simulink model "simulink_tri_motor_drone"  (R2020a)
settings: Solver=VariableStepAuto  StartTime=0.0  StopTime=50  RelTol=1e-3
values from neighbouring files (symbols this model uses):
  airDensity = 1.225    [tri_drone.m]
  areaWheelFront = wheelHeight*wheelWidth    (= 0.004)    [tri_drone.m]
  areaWing = 0.121    [tri_drone.m]
  cDFront = 0.9    [tri_drone.m]
  cDtable = [0.174 0.157 0.141 0.127 0.113 0.100 0.088 0.077 0.067 0.058 0.051 0.044 0.038 0.033 0.028 0.025 0.023 0.021 0.020 0.020 0.021 0.023 0.026 0.029 0.033 0.038 0.043 0.050 0.056 0.064 0.072 0.081 0.091 0.101 0.112 0.124 0.137 0.150 0.165 0.180 0.196 0.212 0.229 0.245 0.261 0.277 0.292 0.306 0.319 0.331 0.341]    [tri_drone.m]
  cLtable = [-1.07 -1.02 -0.97 -0.92 -0.87 -0.81 -0.76 -0.70 -0.65 -0.59 -0.54 -0.48 -0.43 -0.37 -0.31 -0.25 -0.19 -0.13 -0.07 -0.01 0.05 0.11 0.17 0.23 0.29 0.35 0.40 0.46 0.52 0.57 0.63 0.68 0.74 0.79 0.85 0.90 0.95 1.00 1.05 1.10 1.15 1.20 1.25 1.29 1.32 1.36 1.38 1.41 1.43 1.44 1.45]    [tri_drone.m]
  heightRef = 1.0    (= 1)    [tri_drone.m]
  hoverRot = w(11)    [tri_drone.m]
  hoverVel = trustPerPropeller / Ktrust /pi * 180.0    [tri_drone.m]
  hoverVoltagefine = 0.35*11.9    (= 4.165)    [tri_drone.m]
  KDheightcoarse = 15.0    (= 15)    [tri_drone.m]
  KDheightfine = 0    [tri_drone.m]
  KDrag = 8 * (ampMax * Km / (rpmMax / 60 * 2 * pi))    (= 0.000150440801971)    [tri_drone.m]
  KIheightcoarse = 5.0    (= 5)    [tri_drone.m]
  KIheightfine = 0    [tri_drone.m]
  Km = 60/(Kv * 2 * pi)    (= 0.00415186808066)    [tri_drone.m]
  KPheightcoarse = 0.1    [tri_drone.m]
  KPheightfine = 0    [tri_drone.m]
  Ktrust = (trustMax * g)/(rpmMax / 60 * 2 * pi)    (= 0.00223215912077)    [tri_drone.m]
  mBodyTotal = 0.422 + mBattery    (= 0.797)    [tri_drone.m]
  motorMass = 0.022    [tri_drone.m]
  N = 1000000    [tri_drone.m]
  pitch_lower_limit = theta(1)    [tri_drone.m]
  pitch_upper_limit = theta(end)    [tri_drone.m]
  propellerMass = 0.012    [tri_drone.m]
  Ra = RaVolt/ampMax    (= 0.133333333333)    [tri_drone.m]
  rInner = armRadius    (= 0.27)    [tri_drone.m]
  rOuter = armRadius + wLength    (= 0.91)    [tri_drone.m]
  theta = [-10 -9.5 -9.0 -8.5 -8.0 -7.5 -7.0 -6.5 -6.0 -5.5 -5.0 -4.5 -4.0 -3.5 -3.0 -2.5 -2.0 -1.5 -1.0 -0.5 0 0.5 1.0 1.5 2.0 2.5 3.0 3.5 4.0 4.5 5.0 5.5 6.0 6.5 7.0 7.5 8.0 8.5 9.0 9.5 10.0 10.5 11.0 11.5 12.0 12.5 13.0 13.5 14.0 14.5 15.0]    [tri_drone.m]
  Ts = 0.002    [tri_drone.m]
  Ts2 = 0.03    [tri_drone.m]
  wHeight = 0.025    [tri_drone.m]
  wingDensity = 50    [tri_drone.m]
  wLength = 0.64    [tri_drone.m]
  wWidth = 0.20    (= 0.2)    [tri_drone.m]
undefined symbols (not defined in the file or in its folder): X, Y, Z
libraries: sm_lib x53, nesl_utility x45
(part 1 of 3)
settings Model: Creator=Jonas  LastModifiedBy=Jonas

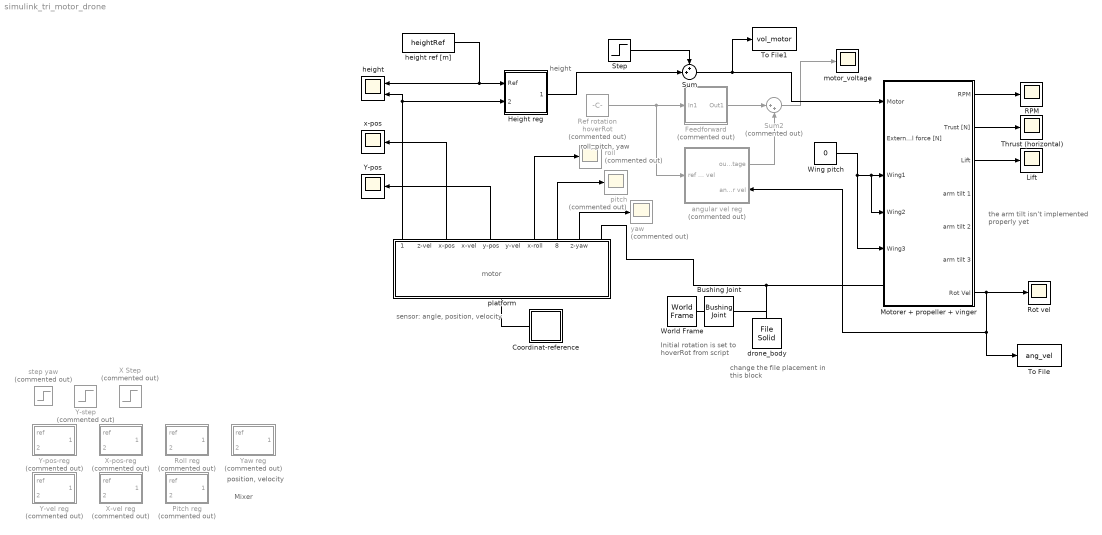
== system simulink_tri_motor_drone ==
  note: the arm tilt isn't implemented properly yet
  note: change the file placement in this block
  note: Initial rotation is set to
      | hoverRot from script
  note: roll, pitch, yaw
  note: position, velocity
  note: height
  note: motor
  note: Mixer
  note: sensor: angle, position, velocity
  Bushing Joint : sm_lib/Joints/Bushing Joint  JointMode=Normal  SenseConstraintForce=off  SenseConstraintForceX=off  SenseConstraintForceY=off  SenseConstraintForceZ=off  SenseConstraintTorque=off  SenseConstraintTorqueX=off  SenseConstraintTorqueY=off  SenseConstraintTorqueZ=off  SenseTotalForce=off  SenseTotalForceX=off  SenseTotalForceY=off  SenseTotalForceZ=off  SenseTotalTorque=off  SenseTotalTorqueX=off  SenseTotalTorqueY=off  SenseTotalTorqueZ=off  CompositeWrenchDir=FollowerOnBase  CompositeWrenchFrame=BaseFrame  PxEquilibriumPosition=0  PxEquilibriumPositionUnits=m  PxSpringStiffness=0  PxSpringStiffnessUnits=N/m  PxDampingCoefficient=0  PxDampingCoefficientUnits=N/(m/s)  PxTorqueActuationMode=NoTorque  PxMotionActuationMode=ComputedMotion  PxSensePosition=off  PxSenseVelocity=off  PxSenseAcceleration=off  PxSenseTorqueForce=off  PxSenseLowerLimitTorqueForce=off  PxSenseUpperLimitTorqueForce=off  PxLowerLimitSpecify=off  PxLowerLimitBound=-1  PxLowerLimitBoundUnits=m  PxLowerLimitStiffness=1e6  PxLowerLimitStiffnessUnits=N/m  PxLowerLimitDamping=1e3  PxLowerLimitDampingUnits=N/(m/s)  PxLowerLimitTransitionRegionWidth=1e-4  PxLowerLimitTransitionRegionWidthUnits=m  PxUpperLimitSpecify=off  PxUpperLimitBound=1  PxUpperLimitBoundUnits=m  PxUpperLimitStiffness=1e6  PxUpperLimitStiffnessUnits=N/m  PxUpperLimitDamping=1e3  PxUpperLimitDampingUnits=N/(m/s)  PxUpperLimitTransitionRegionWidth=1e-4  PxUpperLimitTransitionRegionWidthUnits=m  PxPositionTargetSpecify=off  PxPositionTargetPriority=High  PxPositionTargetValue=0  PxPositionTargetValueUnits=m  PxVelocityTargetSpecify=off  PxVelocityTargetPriority=High  PxVelocityTargetValue=0  PxVelocityTargetValueUnits=m/s  PyEquilibriumPosition=0  PyEquilibriumPositionUnits=m  PySpringStiffness=0  PySpringStiffnessUnits=N/m  PyDampingCoefficient=0  PyDampingCoefficientUnits=N/(m/s)  PyTorqueActuationMode=NoTorque  PyMotionActuationMode=ComputedMotion  PySensePosition=off  PySenseVelocity=off  PySenseAcceleration=off  PySenseTorqueForce=off  PySenseLowerLimitTorqueForce=off  PySenseUpperLimitTorqueForce=off  PyLowerLimitSpecify=off  PyLowerLimitBound=-1  PyLowerLimitBoundUnits=m  PyLowerLimitStiffness=1e6  PyLowerLimitStiffnessUnits=N/m  PyLowerLimitDamping=1e3  PyLowerLimitDampingUnits=N/(m/s)  PyLowerLimitTransitionRegionWidth=1e-4  PyLowerLimitTransitionRegionWidthUnits=m  PyUpperLimitSpecify=off  PyUpperLimitBound=1  PyUpperLimitBoundUnits=m  PyUpperLimitStiffness=1e6  PyUpperLimitStiffnessUnits=N/m  PyUpperLimitDamping=1e3  PyUpperLimitDampingUnits=N/(m/s)  PyUpperLimitTransitionRegionWidth=1e-4  PyUpperLimitTransitionRegionWidthUnits=m  PyPositionTargetSpecify=off  PyPositionTargetPriority=High  PyPositionTargetValue=0  PyPositionTargetValueUnits=m  PyVelocityTargetSpecify=off  PyVelocityTargetPriority=High  PyVelocityTargetValue=0  PyVelocityTargetValueUnits=m/s  PzEquilibriumPosition=0  PzEquilibriumPositionUnits=m  PzSpringStiffness=0  PzSpringStiffnessUnits=N/m  PzDampingCoefficient=0  PzDampingCoefficientUnits=N/(m/s)  PzTorqueActuationMode=NoTorque  PzMotionActuationMode=ComputedMotion  PzSensePosition=off  PzSenseVelocity=off  PzSenseAcceleration=off  PzSenseTorqueForce=off  PzSenseLowerLimitTorqueForce=off  PzSenseUpperLimitTorqueForce=off  PzLowerLimitSpecify=off  PzLowerLimitBound=-1  PzLowerLimitBoundUnits=m  PzLowerLimitStiffness=1e6  PzLowerLimitStiffnessUnits=N/m  PzLowerLimitDamping=1e3  PzLowerLimitDampingUnits=N/(m/s)  PzLowerLimitTransitionRegionWidth=1e-4  PzLowerLimitTransitionRegionWidthUnits=m  PzUpperLimitSpecify=off  PzUpperLimitBound=1  PzUpperLimitBoundUnits=m  PzUpperLimitStiffness=1e6  PzUpperLimitStiffnessUnits=N/m  PzUpperLimitDamping=1e3  PzUpperLimitDampingUnits=N/(m/s)  PzUpperLimitTransitionRegionWidth=1e-4  PzUpperLimitTransitionRegionWidthUnits=m  PzPositionTargetSpecify=off  PzPositionTargetPriority=High  PzPositionTargetValue=0  PzPositionTargetValueUnits=m  PzVelocityTargetSpecify=off  PzVelocityTargetPriority=High  PzVelocityTargetValue=0  PzVelocityTargetValueUnits=m/s  RxEquilibriumPosition=0  RxEquilibriumPositionUnits=deg  RxSpringStiffness=0  RxSpringStiffnessUnits=N*m/deg  RxDampingCoefficient=0  RxDampingCoefficientUnits=N*m/(deg/s)  RxTorqueActuationMode=NoTorque  RxMotionActuationMode=ComputedMotion  RxSensePosition=off  RxSenseVelocity=off  RxSenseAcceleration=off  RxSenseTorqueForce=off  RxSenseLowerLimitTorqueForce=off  RxSenseUpperLimitTorqueForce=off  RxLowerLimitSpecify=off  RxLowerLimitBound=-90  RxLowerLimitBoundUnits=deg  RxLowerLimitStiffness=1e4  RxLowerLimitStiffnessUnits=N*m/deg  RxLowerLimitDamping=10  RxLowerLimitDampingUnits=N*m/(deg/s)  RxLowerLimitTransitionRegionWidth=0.1  RxLowerLimitTransitionRegionWidthUnits=deg  RxUpperLimitSpecify=off  RxUpperLimitBound=90  RxUpperLimitBoundUnits=deg  RxUpperLimitStiffness=1e4  RxUpperLimitStiffnessUnits=N*m/deg  RxUpperLimitDamping=10  RxUpperLimitDampingUnits=N*m/(deg/s)  RxUpperLimitTransitionRegionWidth=0.1  RxUpperLimitTransitionRegionWidthUnits=deg  RxPositionTargetSpecify=off  RxPositionTargetPriority=High  RxPositionTargetValue=0  RxPositionTargetValueUnits=deg  RxVelocityTargetSpecify=off  RxVelocityTargetPriority=High  RxVelocityTargetValue=0  RxVelocityTargetValueUnits=deg/s  RyEquilibriumPosition=0  RyEquilibriumPositionUnits=deg  RySpringStiffness=0  RySpringStiffnessUnits=N*m/deg  RyDampingCoefficient=0  RyDampingCoefficientUnits=N*m/(deg/s)  RyTorqueActuationMode=NoTorque  RyMotionActuationMode=ComputedMotion  RySensePosition=off  RySenseVelocity=off  RySenseAcceleration=off  RySenseTorqueForce=off  RySenseLowerLimitTorqueForce=off  RySenseUpperLimitTorqueForce=off  RyLowerLimitSpecify=off  RyLowerLimitBound=-90  RyLowerLimitBoundUnits=deg  RyLowerLimitStiffness=1e4  RyLowerLimitStiffnessUnits=N*m/deg  RyLowerLimitDamping=10  RyLowerLimitDampingUnits=N*m/(deg/s)  RyLowerLimitTransitionRegionWidth=0.1  RyLowerLimitTransitionRegionWidthUnits=deg  RyUpperLimitSpecify=off  RyUpperLimitBound=90  RyUpperLimitBoundUnits=deg  RyUpperLimitStiffness=1e4  RyUpperLimitStiffnessUnits=N*m/deg  RyUpperLimitDamping=10  RyUpperLimitDampingUnits=N*m/(deg/s)  RyUpperLimitTransitionRegionWidth=0.1  RyUpperLimitTransitionRegionWidthUnits=deg  RyPositionTargetSpecify=off  RyPositionTargetPriority=High  RyPositionTargetValue=0  RyPositionTargetValueUnits=deg  RyVelocityTargetSpecify=off  RyVelocityTargetPriority=High  RyVelocityTargetValue=0  RyVelocityTargetValueUnits=deg/s  RzEquilibriumPosition=0  RzEquilibriumPositionUnits=deg  RzSpringStiffness=0  RzSpringStiffnessUnits=N*m/deg  RzDampingCoefficient=0  RzDampingCoefficientUnits=N*m/(deg/s)  RzTorqueActuationMode=NoTorque  RzMotionActuationMode=ComputedMotion  RzSensePosition=off  RzSenseVelocity=off  RzSenseAcceleration=off  RzSenseTorqueForce=off  RzSenseLowerLimitTorqueForce=off  RzSenseUpperLimitTorqueForce=off  RzLowerLimitSpecify=off  RzLowerLimitBound=-90  RzLowerLimitBoundUnits=deg  RzLowerLimitStiffness=1e4  RzLowerLimitStiffnessUnits=N*m/deg  RzLowerLimitDamping=10  RzLowerLimitDampingUnits=N*m/(deg/s)  RzLowerLimitTransitionRegionWidth=0.1  RzLowerLimitTransitionRegionWidthUnits=deg  RzUpperLimitSpecify=off  RzUpperLimitBound=90  RzUpperLimitBoundUnits=deg  RzUpperLimitStiffness=1e4  RzUpperLimitStiffnessUnits=N*m/deg  RzUpperLimitDamping=10  RzUpperLimitDampingUnits=N*m/(deg/s)  RzUpperLimitTransitionRegionWidth=0.1  RzUpperLimitTransitionRegionWidthUnits=deg  RzPositionTargetSpecify=off  RzPositionTargetPriority=High  RzPositionTargetValue=0  RzPositionTargetValueUnits=deg  RzVelocityTargetSpecify=on  RzVelocityTargetPriority=High  RzVelocityTargetValue=initRot  RzVelocityTargetValueUnits=rad/s
  Coordinat-reference : Subsystem
  Feedforward : Subsystem  Commented=on
  Height reg : Subsystem
  Lift : Scope
  Motorer + propeller + vinger : Subsystem
  Pitch reg : Subsystem  Commented=on
  RPM : Scope
  Ref rotation : Constant  Commented=on  Value=hoverRot
  Roll reg : Subsystem  Commented=on
  Rot vel : Scope
  Step : Step  Time=25  After=0.39*11.9  SampleTime=0
  Sum : Sum  Inputs=++|
  Sum2 : Sum  Commented=on  Inputs=|++
  Thrust (horizontal) : Scope
  To File : ToFile  Filename=ang_vel
  To File1 : ToFile  Filename=vol_motor
  Wing pitch : Constant  Value=0
  World Frame : sm_lib/Frames and Transforms/World Frame
  X Step : Step  Commented=on  Time=1.5  After=0  SampleTime=0
  X-pos-reg : Subsystem  Commented=on
  X-vel reg : Subsystem  Commented=on
  Y-pos : Scope
  Y-pos-reg : Subsystem  Commented=on
  Y-step : Step  Commented=on  After=0  SampleTime=0
  Y-vel reg : Subsystem  Commented=on
  "Yaw reg " : Subsystem  Commented=on
  angular vel reg : Subsystem  Commented=on
      settings: PortSchema="{\"entries\":[{\"content\":{\"sides\":[{\"content\":{\"connectorIds\":[\"In1\"]},\"type\":\"ConnectorPlacement.EquallySpacedRectSide\",\"uuid\":\"77c843f2-849e-4254-8ab0-e659ee2bffc0\"},{\"content\":{\"connectorIds\":[\"Out1\",\"In2\"],\"side\":\"RIGHT\"},\"type\":\"ConnectorPlacement.EquallySpacedRectSide\",\"uuid\":\"827c0fe3-5880-493e-8320-005b0a787497\"},{\"content\":{\"connectorIds\":[],\"side\":\"TOP\"},\"type\":\"ConnectorPlacement.EquallySpacedRectSide\",\"uuid\":\"d374b84c-e282-483e-a15b-002a2b8dff42\"}]},\"type\":\"ConnectorPlacement.EquallySpacedConnector\",\"uuid\":\"ceb3a894-fc48-462a-be70-379008192682\"}],\"packageUris\":[\"http://schema.mathworks.com/mf0/Connector/19700101\"],\"version\":\"1.0\"}"
  drone_body : sm_lib/Body Elements/File Solid  Tag=drone_body  ExtGeomFileName=C:\Sync\Dokumenter\Universitet\6_Semester\Bachelorprojekt\solidworks (3dmodel)\drone3d.SLDPRT  UnitType=FromFile  ExtGeomFileUnits=m  StepReaderType=HEX  ExportConvexHullGeometry=off  InertiaType=CalculateFromGeometry  Mass=mBodyTotal  MassUnits=kg  CenterOfMass=[0 0 0]  CenterOfMassUnits=m  MomentsOfInertia=[1 1 1]  MomentsOfInertiaUnits=kg*m^2  ProductsOfInertia=[0 0 0]  ProductsOfInertiaUnits=kg*m^2  BasedOnType=Mass  Density=1000  DensityUnits=kg/m^3  DoExposeReferenceFrame=on  SerializedFrames=<Frames/>  GraphicType=FromGeometry  MarkerShape=Sphere  MarkerSize=10  GraphicVisPropType=SimpleVisualProperties  GraphicDiffuseColor=[0.5 0.5 0.5]  GraphicSpecularColor=[0.5 0.5 0.5 1.0]  GraphicAmbientColor=[0.15 0.15 0.15 1.0]  GraphicEmissiveColor=[0.0 0.0 0.0 1.0]  GraphicShininess=75  GraphicOpacity=1.0
  height : Scope  NumInputPorts=2
  height ref [m] : Constant  Value=heightRef
  motor_voltage : Scope
  pitch : Scope  Commented=on
  platform : Subsystem
  roll : Scope  Commented=on
  step yaw : Step  Commented=on  Time=2  After=0  SampleTime=0
  x-pos : Scope
  yaw : Scope  Commented=on
  wires:
  platform/3(x-pos) -> x-pos/1
  platform/8(y-pitch) -> pitch/1
  platform/9(z-yaw) -> yaw/1
  platform/5(y-pos) -> Y-pos/1
  Motorer + propeller + vinger/1(RPM) -> RPM/1
  platform/7(x-roll) -> roll/1
  platform/1(Drone z-pos) -> height/2, Height reg/2(Measured)
  Motorer + propeller + vinger/3(Lift) -> Lift/1
  Motorer + propeller + vinger/2(Trust [N]) -> Thrust (horizontal)/1
  height ref [m]/1 -> height/1, Height reg/1(Ref)
  Motorer + propeller + vinger/7(Rot Vel) -> Rot vel/1, To File/1, angular vel reg/2(angular vel)
  Ref rotation/1 -> angular vel reg/1(ref ang vel), Feedforward/1(In1)
  angular vel reg/1(output voltage) -> Sum2/2
  Sum2/1 -> motor_voltage/1
  Feedforward/1(Out1) -> Sum2/1
  Wing pitch/1 -> Motorer + propeller + vinger/5(Wing3), Motorer + propeller + vinger/4(Wing2), Motorer + propeller + vinger/3(Wing1)
  Height reg/1(u-trust) -> Sum/2
  Step/1 -> Sum/1
  Sum/1 -> To File1/1, Motorer + propeller + vinger/1(Motor)
  connections:
  platform/RConn1 -- Bushing Joint/RConn1 -- drone_body/RConn1 -- Motorer + propeller + vinger/LConn1
  platform/LConn1 -- Coordinat-reference/RConn1
  Bushing Joint/LConn1 -- World Frame/RConn1

== system simulink_tri_motor_drone/Coordinat-reference ==
  Mechanism Configuration : sm_lib/Utilities/Mechanism Configuration  UniformGravity=Constant  GravityVector=[0 0 -9.80665]  GravityUnits=m/s^2  LinearizationDelta=0.001
  Solver Configuration : nesl_utility/Solver Configuration  PhysicalDomain=network_engine_domain  SubClassName=solver  LeftPortType=input  RightPortType=generic  Tones=[]  Harmonics=[]  SimulateNoise=off  Profile=off  UseLocalSampling=off  EnableSwitchedLinearOptims=on  FrequencyDomain=off  UseCCode=off  RelTol=0.001  AbsTol=1e-06  MinStep=1e-09  ToWorkspace=off  RevertToSquareIcSolve=off  NumHomotopyIterations=100  PhasorMode=off  PhasorModeNumHarmonics=1  DoDC=off  ResidualTolerance=1e-09  UseLocalSolver=off  LocalSolverChoice=NE_BACKWARD_EULER_ADVANCER  LocalSolverSampleTime=0.001  DoFixedCost=off  MaxNonlinIter=3  MaxModeIter=2  LinearAlgebra=Sparse  EquationFormulation=NE_TIME_EF  DelaysMemoryBudget=1024  AutomaticFiltering=on  FilteringTimeConstant=0.001  PartitionStorageMethod=AS_NEEDED  PartitionMemoryBudget=1024  PartitionMethod=FAST
  World Frame : sm_lib/Frames and Transforms/World Frame
  ground : sm_lib/Body Elements/Brick Solid  GraphicAmbientColor=[0.15 0.15 0.15 1.0]  BasedOnType=Mass  BrickDimensions=[1 1 0.01]  BrickDimensionUnits=m  CenterOfMass=[0 0 0]  CenterOfMassUnits=m  GraphicDiffuseColor=[0.2 0.5 0.2]  Density=1000  DensityUnits=kg/(m^3)  DoExposeReferenceFrame=on  GraphicEmissiveColor=[0.0 0.0 0.0 1.0]  ExportEntireGeometry=off  SerializedFrames=<Frames/>  MarkerShape=Sphere  MarkerSize=10  GraphicType=FromGeometry  InertiaType=CalculateFromGeometry  Mass=1  MassUnits=kg  MomentsOfInertia=[1 1 1]  MomentsOfInertiaUnits=kg*m^2  GraphicOpacity=1.0  ProductsOfInertia=[0 0 0]  ProductsOfInertiaUnits=kg*m^2  GraphicShininess=75  GraphicSpecularColor=[0.5 0.5 0.5 1.0]  GraphicVisPropType=SimpleVisualProperties
  Conn1 : PMIOPort  Side=Right
  connections:
  Solver Configuration/RConn1 -- Conn1/RConn1 -- ground/RConn1 -- World Frame/RConn1 -- Mechanism Configuration/RConn1

== system simulink_tri_motor_drone/Feedforward ==
  In1 : Inport
  Constant : Constant  Commented=on  Value=66005
  Constant1 : Constant  Value=4.164519326
  Gain : Gain  Gain=0.4955401388
  Gain1 : Gain  Commented=through  Gain=0.04
  Sqrt : Sqrt  Commented=through  SaturateOnIntegerOverflow=on
  Sqrt1 : Sqrt  Commented=through  SaturateOnIntegerOverflow=on
  Sum : Sum  Inputs=|++
  Sum1 : Sum  Inputs=|-+
  Out1 : Outport
  wires:
  In1/1 -> Sqrt/1
  Sqrt/1 -> Gain/1
  Gain/1 -> Sum/2
  Constant/1 -> Sum/1
  Sum/1 -> Sqrt1/1
  Gain1/1 -> Sum1/2
  Constant1/1 -> Sum1/1
  Sum1/1 -> Out1/1
  Sqrt1/1 -> Gain1/1

== system simulink_tri_motor_drone/Height reg ==
  Ref : Inport
  Measured : Inport  Port=2
  Coarse controller (>5m error) : Subsystem  Commented=on  TreatAsAtomicUnit=on
  Constant : Constant  Commented=on
  Constant1 : Constant  Value=hoverVoltagefine
  Fine controller (<5m error) : Subsystem  Commented=on  TreatAsAtomicUnit=on
  If : If  Commented=on  IfExpression=u1 > 5
  KD : Constant  Value=KDheightfine
  KI : Constant  Value=KIheightfine
  KP : Constant  Value=KPheightfine
  Rate Transition : RateTransition  Commented=on  OutPortSampleTime=Ts
  Sum : Sum  Inputs=|+-
  Sum1 : Sum  Inputs=|++
  height-controller-fine : Subsystem
  height-error : Scope
  u-trust : Outport
  wires:
  Measured/1 -> Sum/2
  Ref/1 -> Sum/1
  Sum/1 -> height-controller-fine/4(fejl), height-error/1, Coarse controller (>5m error)/1(fejl), Fine controller (<5m error)/1(fejl)
  If/1 -> Coarse controller (>5m error)/Action
  If/2 -> Fine controller (<5m error)/Action
  Constant/1 -> Rate Transition/1
  Rate Transition/1 -> If/1
  KD/1 -> height-controller-fine/2(KD)
  KI/1 -> height-controller-fine/1(KI)
  KP/1 -> height-controller-fine/3(KP)
  height-controller-fine/1(Out1) -> Sum1/1
  Constant1/1 -> Sum1/2
  Sum1/1 -> u-trust/1

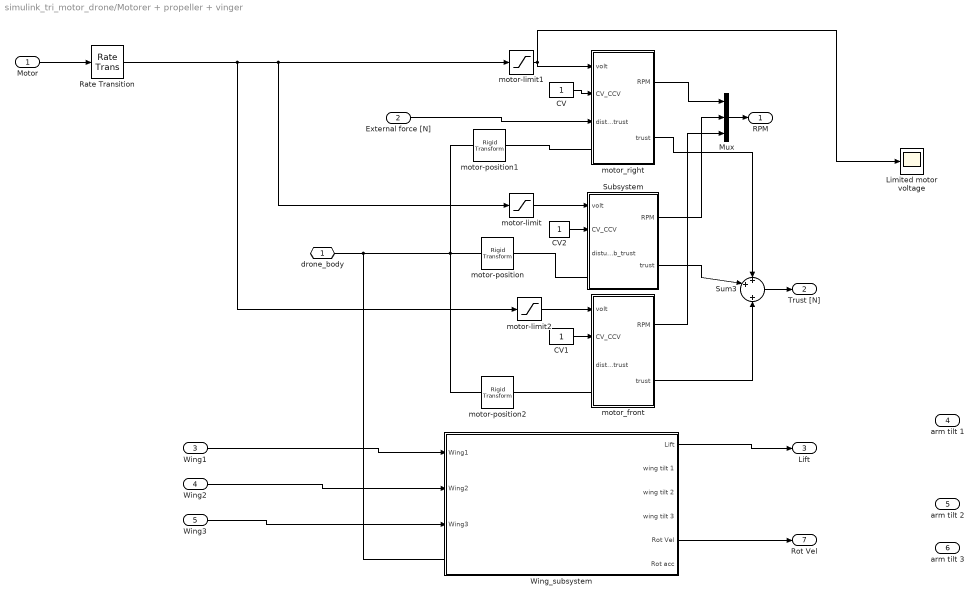
== system simulink_tri_motor_drone/Motorer + propeller + vinger ==
  Motor : Inport
  External force [N] : Inport  Port=2
  Wing1 : Inport  Port=3
  Wing2 : Inport  Port=4
  Wing3 : Inport  Port=5
  CV : Constant
  CV1 : Constant
  CV2 : Constant
  Limited motor voltage : Scope
  Mux : Mux  Inputs=3
  Rate Transition : RateTransition  OutPortSampleTime=0.1
  Subsystem : Subsystem
  Sum3 : Sum  Inputs=++|+
  Wing_subsystem : Subsystem
  motor-limit : Saturate  UpperLimit=11  LowerLimit=0
  motor-limit1 : Saturate  UpperLimit=11  LowerLimit=0
  motor-limit2 : Saturate  UpperLimit=11  LowerLimit=0
  motor-position : sm_lib/Frames and Transforms/Rigid Transform  TranslationMethod=Cartesian  TranslationStandardOffset=0  TranslationLengthUnit=m  TranslationStandardAxis=+Z  TranslationCartesianOffset=offSet2  TranslationROffset=0.27  TranslationROffsetUnits=m  TranslationZOffset=0  TranslationZOffsetUnits=m  TranslationThetaOffset=0  TranslationThetaOffsetUnits=deg  RotationMethod=RotationSequence  RotationAngleUnits=deg  RotationStandardAxis=+Y  RotationAngle=90  RotationArbitraryAxis=[0 0 1]  FollAlignAxisA=+X  BaseAlignAxisA=+Y  FollAlignAxisB=+Y  BaseAlignAxisB=+Z  RotationSequenceAxes=BaseAxes  RotationSequence=XYZ  RotationSequenceAngles=[-90 0 120]  RotationSequenceAnglesUnits=deg  RotationMatrix=[1 0 0; 0 1 0; 0 0 1]
  motor-position1 : sm_lib/Frames and Transforms/Rigid Transform  TranslationMethod=Cartesian  TranslationStandardOffset=0  TranslationLengthUnit=m  TranslationStandardAxis=+Z  TranslationCartesianOffset=offSet1  TranslationROffset=0.27  TranslationROffsetUnits=m  TranslationZOffset=0  TranslationZOffsetUnits=m  TranslationThetaOffset=0  TranslationThetaOffsetUnits=deg  RotationMethod=RotationSequence  RotationAngleUnits=deg  RotationStandardAxis=+Y  RotationAngle=90  RotationArbitraryAxis=[0 0 1]  FollAlignAxisA=+X  BaseAlignAxisA=+Y  FollAlignAxisB=+Y  BaseAlignAxisB=+Z  RotationSequenceAxes=BaseAxes  RotationSequence=XYZ  RotationSequenceAngles=[-90 0 0]  RotationSequenceAnglesUnits=deg  RotationMatrix=[1 0 0; 0 1 0; 0 0 1]
  motor-position2 : sm_lib/Frames and Transforms/Rigid Transform  TranslationMethod=Cartesian  TranslationStandardOffset=0  TranslationLengthUnit=m  TranslationStandardAxis=+Z  TranslationCartesianOffset=offSet3  TranslationROffset=0.27  TranslationROffsetUnits=m  TranslationZOffset=0  TranslationZOffsetUnits=m  TranslationThetaOffset=0  TranslationThetaOffsetUnits=deg  RotationMethod=RotationSequence  RotationAngleUnits=deg  RotationStandardAxis=+Y  RotationAngle=90  RotationArbitraryAxis=[0 0 1]  FollAlignAxisA=+X  BaseAlignAxisA=+Y  FollAlignAxisB=+Y  BaseAlignAxisB=+Z  RotationSequenceAxes=BaseAxes  RotationSequence=XYZ  RotationSequenceAngles=[-90 0 240]  RotationSequenceAnglesUnits=deg  RotationMatrix=[1 0 0; 0 1 0; 0 0 1]
  motor_front : Subsystem
  motor_right : Subsystem
  drone_body : PMIOPort  Side=Left
  RPM : Outport  VectorParamsAs1DForOutWhenUnconnected=off
  Trust [N] : Outport  Port=2  VectorParamsAs1DForOutWhenUnconnected=off
  Lift : Outport  Port=3
  arm tilt 1 : Outport  Port=4
  arm tilt 2 : Outport  Port=5
  arm tilt 3 : Outport  Port=6
  Rot Vel : Outport  Port=7
  wires:
  External force [N]/1 -> motor_right/3(disturb_trust)
  motor_right/2(trust) -> Sum3/1
  Subsystem/2(trust) -> Sum3/2
  CV/1 -> motor_right/2(CV_CCV)
  CV2/1 -> Subsystem/2(CV_CCV)
  Mux/1 -> RPM/1
  Sum3/1 -> Trust [N]/1
  motor-limit/1 -> Subsystem/1(volt)
  Subsystem/1(RPM) -> Mux/2
  Motor/1 -> Rate Transition/1
  motor-limit2/1 -> motor_front/1(volt)
  CV1/1 -> motor_front/2(CV_CCV)
  motor_front/2(trust) -> Sum3/3
  motor_front/1(RPM) -> Mux/3
  motor_right/1(RPM) -> Mux/1
  Wing3/1 -> Wing_subsystem/3(Wing3)
  Wing2/1 -> Wing_subsystem/2(Wing2)
  Wing1/1 -> Wing_subsystem/1(Wing1)
  Wing_subsystem/1(Lift) -> Lift/1
  motor-limit1/1 -> motor_right/1(volt), Limited motor voltage/1
  Wing_subsystem/5(Rot Vel) -> Rot Vel/1
  Rate Transition/1 -> motor-limit2/1, motor-limit/1, motor-limit1/1
  connections:
  motor-position1/RConn1 -- motor_right/LConn1
  motor-position/RConn1 -- Subsystem/LConn1
  motor-position2/RConn1 -- motor_front/LConn1
  motor-position/LConn1 -- Wing_subsystem/LConn1 -- drone_body/RConn1 -- motor-position2/LConn1 -- motor-position1/LConn1

== system simulink_tri_motor_drone/Pitch reg ==
  ref : Inport
  measured : Inport  Port=2
  KDr : Constant  Value=0.5
  KIr : Constant
  KPr : Constant  Value=0.8
  Pitch-u : Scope
  pitch-controller : Subsystem
  pitch_rad : Scope
  u - pitch : Outport  VectorParamsAs1DForOutWhenUnconnected=off
  wires:
  ref/1 -> pitch-controller/5(ref)
  KDr/1 -> pitch-controller/2(KD)
  KPr/1 -> pitch-controller/3(KP)
  measured/1 -> pitch_rad/1, pitch-controller/4(measured)
  pitch-controller/1(Out1) -> Pitch-u/1, u - pitch/1
  KIr/1 -> pitch-controller/1(KI)

== system simulink_tri_motor_drone/Roll reg ==
  ref : Inport
  measured : Inport  Port=2
  KDr : Constant  Value=0.5
  KIr : Constant
  KPr : Constant  Value=0.8
  Roll-u : Scope
  Roll_rad : Scope
  roll-controller : Subsystem
  u-roll : Outport  VectorParamsAs1DForOutWhenUnconnected=off
  wires:
  KIr/1 -> roll-controller/1(KI)
  roll-controller/1(Out1) -> u-roll/1, Roll-u/1
  measured/1 -> roll-controller/4(measured), Roll_rad/1
  KPr/1 -> roll-controller/3(KP)
  KDr/1 -> roll-controller/2(KD)
  ref/1 -> roll-controller/5(ref)

== system simulink_tri_motor_drone/X-pos-reg ==
  ref : Inport
  measured : Inport  Port=2
  KDr : Constant  Value=0.00015
  KIr : Constant  Value=0
  KPr : Constant
  Saturation : Saturate  UpperLimit=1  LowerLimit=-1
  X-pos-u : Scope
  x-pos-controller : Subsystem
  u - pitch : Outport  VectorParamsAs1DForOutWhenUnconnected=off
  wires:
  KIr/1 -> x-pos-controller/1(KI)
  x-pos-controller/1(Out1) -> Saturation/1
  measured/1 -> x-pos-controller/4(measured)
  KPr/1 -> x-pos-controller/3(KP)
  KDr/1 -> x-pos-controller/2(KD)
  ref/1 -> x-pos-controller/5(ref)
  Saturation/1 -> u - pitch/1, X-pos-u/1

== system simulink_tri_motor_drone/X-vel reg ==
  ref : Inport
  measured : Inport  Port=2
  KDr : Constant  Value=0.1
  KIr : Constant  Value=0
  KPr : Constant  Value=0.08
  Saturation : Saturate  UpperLimit=0.05  LowerLimit=-0.05
  X-vel-u : Scope
  x-vel-controller : Subsystem
  u - pitch : Outport  VectorParamsAs1DForOutWhenUnconnected=off
  wires:
  Saturation/1 -> X-vel-u/1, u - pitch/1
  ref/1 -> x-vel-controller/5(ref)
  KDr/1 -> x-vel-controller/2(KD)
  KPr/1 -> x-vel-controller/3(KP)
  measured/1 -> x-vel-controller/4(measured)
  x-vel-controller/1(Out1) -> Saturation/1
  KIr/1 -> x-vel-controller/1(KI)

== system simulink_tri_motor_drone/Y-pos-reg ==
  ref : Inport
  measured : Inport  Port=2
  KDr : Constant  Value=0.00015
  KIr : Constant  Value=0
  KPr : Constant
  Saturation : Saturate  UpperLimit=1  LowerLimit=-1
  Y-pos-controller : Subsystem
  Y-pos-u : Scope
  u - pitch : Outport  VectorParamsAs1DForOutWhenUnconnected=off
  wires:
  Saturation/1 -> Y-pos-u/1, u - pitch/1
  ref/1 -> Y-pos-controller/5(ref)
  KDr/1 -> Y-pos-controller/2(KD)
  KPr/1 -> Y-pos-controller/3(KP)
  measured/1 -> Y-pos-controller/4(measured)
  Y-pos-controller/1(Out1) -> Saturation/1
  KIr/1 -> Y-pos-controller/1(KI)

== system simulink_tri_motor_drone/Y-vel reg ==
  ref : Inport
  measured : Inport  Port=2
  KDr : Constant  Value=0.1
  KIr : Constant  Value=0
  KPr : Constant  Value=0.08
  Saturation : Saturate  UpperLimit=0.05  LowerLimit=-0.05
  Y-vel-controller : Subsystem
  Y-vel-u : Scope
  u - pitch : Outport  VectorParamsAs1DForOutWhenUnconnected=off
  wires:
  KIr/1 -> Y-vel-controller/1(KI)
  Y-vel-controller/1(Out1) -> Saturation/1
  measured/1 -> Y-vel-controller/4(measured)
  KPr/1 -> Y-vel-controller/3(KP)
  KDr/1 -> Y-vel-controller/2(KD)
  ref/1 -> Y-vel-controller/5(ref)
  Saturation/1 -> u - pitch/1, Y-vel-u/1

== system simulink_tri_motor_drone/Yaw reg  ==
  ref : Inport
  measured : Inport  Port=2
  KDr : Constant  Value=0.15
  KIr : Constant  Value=0
  KPr : Constant  Value=10
  Saturation : Saturate
  Yaw-controller : Subsystem
  Yaw-u : Scope
  Yaw_rad : Scope
  u - yaw : Outport  VectorParamsAs1DForOutWhenUnconnected=off
  wires:
  KIr/1 -> Yaw-controller/1(KI)
  Yaw-controller/1(Out1) -> Saturation/1
  measured/1 -> Yaw-controller/4(measured), Yaw_rad/1
  KPr/1 -> Yaw-controller/3(KP)
  KDr/1 -> Yaw-controller/2(KD)
  ref/1 -> Yaw-controller/5(ref)
  Saturation/1 -> u - yaw/1, Yaw-u/1

== system simulink_tri_motor_drone/angular vel reg ==
  ref ang vel : Inport
  angular vel : Inport  Port=2
  KD : Constant  Value=1.1
  KI : Constant  Value=0
  KP : Constant  Value=1.5
  Sum : Sum  Inputs=|+-
  angle_vel error : Scope
  angle_vel_controller : Subsystem
  output voltage : Outport  VectorParamsAs1DForOutWhenUnconnected=off
  wires:
  angular vel/1 -> Sum/2
  ref ang vel/1 -> Sum/1
  angle_vel_controller/1(Out1) -> output voltage/1
  Sum/1 -> angle_vel error/1, angle_vel_controller/4(fejl)
  KP/1 -> angle_vel_controller/3(KP)
  KD/1 -> angle_vel_controller/2(KD)
  KI/1 -> angle_vel_controller/1(KI)

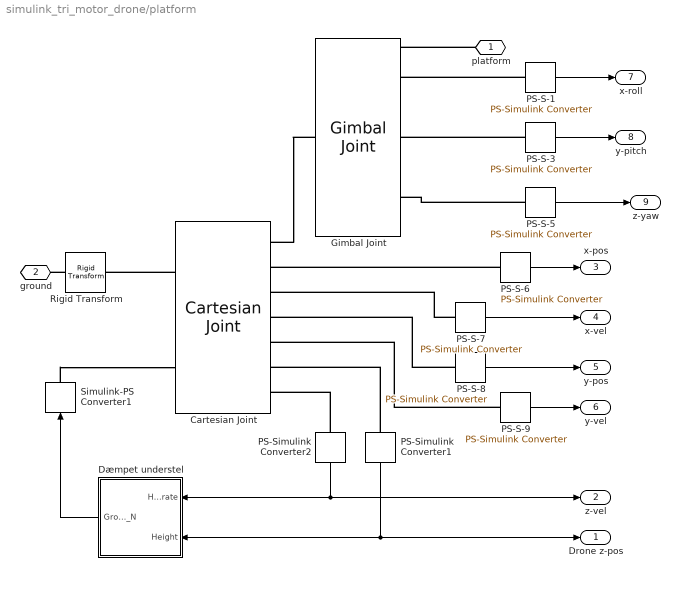
== system simulink_tri_motor_drone/platform ==
  Cartesian Joint : sm_lib/Joints/Cartesian Joint  JointMode=Normal  SenseConstraintForce=off  SenseConstraintForceX=off  SenseConstraintForceY=off  SenseConstraintForceZ=off  SenseConstraintTorque=off  SenseConstraintTorqueX=off  SenseConstraintTorqueY=off  SenseConstraintTorqueZ=off  SenseTotalForce=off  SenseTotalForceX=off  SenseTotalForceY=off  SenseTotalForceZ=off  SenseTotalTorque=off  SenseTotalTorqueX=off  SenseTotalTorqueY=off  SenseTotalTorqueZ=off  CompositeWrenchDir=FollowerOnBase  CompositeWrenchFrame=BaseFrame  PxEquilibriumPosition=0  PxEquilibriumPositionUnits=m  PxSpringStiffness=0  PxSpringStiffnessUnits=N/m  PxDampingCoefficient=0  PxDampingCoefficientUnits=N/(m/s)  PxTorqueActuationMode=NoTorque  PxMotionActuationMode=ComputedMotion  PxSensePosition=on  PxSenseVelocity=on  PxSenseAcceleration=off  PxSenseTorqueForce=off  PxSenseLowerLimitTorqueForce=off  PxSenseUpperLimitTorqueForce=off  PxLowerLimitSpecify=off  PxLowerLimitBound=-1  PxLowerLimitBoundUnits=m  PxLowerLimitStiffness=1e6  PxLowerLimitStiffnessUnits=N/m  PxLowerLimitDamping=1e3  PxLowerLimitDampingUnits=N/(m/s)  PxLowerLimitTransitionRegionWidth=1e-4  PxLowerLimitTransitionRegionWidthUnits=m  PxUpperLimitSpecify=off  PxUpperLimitBound=1  PxUpperLimitBoundUnits=m  PxUpperLimitStiffness=1e6  PxUpperLimitStiffnessUnits=N/m  PxUpperLimitDamping=1e3  PxUpperLimitDampingUnits=N/(m/s)  PxUpperLimitTransitionRegionWidth=1e-4  PxUpperLimitTransitionRegionWidthUnits=m  PxPositionTargetSpecify=off  PxPositionTargetPriority=High  PxPositionTargetValue=0  PxPositionTargetValueUnits=m  PxVelocityTargetSpecify=off  PxVelocityTargetPriority=High  PxVelocityTargetValue=0  PxVelocityTargetValueUnits=m/s  PyEquilibriumPosition=0  PyEquilibriumPositionUnits=m  PySpringStiffness=0  PySpringStiffnessUnits=N/m  PyDampingCoefficient=0  PyDampingCoefficientUnits=N/(m/s)  PyTorqueActuationMode=NoTorque  PyMotionActuationMode=ComputedMotion  PySensePosition=on  PySenseVelocity=on  PySenseAcceleration=off  PySenseTorqueForce=off  PySenseLowerLimitTorqueForce=off  PySenseUpperLimitTorqueForce=off  PyLowerLimitSpecify=off  PyLowerLimitBound=-1  PyLowerLimitBoundUnits=m  PyLowerLimitStiffness=1e6  PyLowerLimitStiffnessUnits=N/m  PyLowerLimitDamping=1e3  PyLowerLimitDampingUnits=N/(m/s)  PyLowerLimitTransitionRegionWidth=1e-4  PyLowerLimitTransitionRegionWidthUnits=m  PyUpperLimitSpecify=off  PyUpperLimitBound=1  PyUpperLimitBoundUnits=m  PyUpperLimitStiffness=1e6  PyUpperLimitStiffnessUnits=N/m  PyUpperLimitDamping=1e3  PyUpperLimitDampingUnits=N/(m/s)  PyUpperLimitTransitionRegionWidth=1e-4  PyUpperLimitTransitionRegionWidthUnits=m  PyPositionTargetSpecify=off  PyPositionTargetPriority=High  PyPositionTargetValue=0  PyPositionTargetValueUnits=m  PyVelocityTargetSpecify=off  PyVelocityTargetPriority=High  PyVelocityTargetValue=0  PyVelocityTargetValueUnits=m/s  PzEquilibriumPosition=0  PzEquilibriumPositionUnits=m  PzSpringStiffness=0  PzSpringStiffnessUnits=N/m  PzDampingCoefficient=0  PzDampingCoefficientUnits=N/(m/s)  PzTorqueActuationMode=InputTorque  PzMotionActuationMode=ComputedMotion  PzSensePosition=on  PzSenseVelocity=on  PzSenseAcceleration=off  PzSenseTorqueForce=off  PzSenseLowerLimitTorqueForce=off  PzSenseUpperLimitTorqueForce=off  PzLowerLimitSpecify=off  PzLowerLimitBound=-1  PzLowerLimitBoundUnits=m  PzLowerLimitStiffness=1e6  PzLowerLimitStiffnessUnits=N/m  PzLowerLimitDamping=1e3  PzLowerLimitDampingUnits=N/(m/s)  PzLowerLimitTransitionRegionWidth=1e-4  PzLowerLimitTransitionRegionWidthUnits=m  PzUpperLimitSpecify=off  PzUpperLimitBound=1  PzUpperLimitBoundUnits=m  PzUpperLimitStiffness=1e6  PzUpperLimitStiffnessUnits=N/m  PzUpperLimitDamping=1e3  PzUpperLimitDampingUnits=N/(m/s)  PzUpperLimitTransitionRegionWidth=1e-4  PzUpperLimitTransitionRegionWidthUnits=m  PzPositionTargetSpecify=on  PzPositionTargetPriority=High  PzPositionTargetValue=heightDeploy  PzPositionTargetValueUnits=m  PzVelocityTargetSpecify=off  PzVelocityTargetPriority=High  PzVelocityTargetValue=0  PzVelocityTargetValueUnits=m/s
  Dæmpet understel : Subsystem
  Gimbal Joint : sm_lib/Joints/Gimbal Joint  JointMode=Normal  SenseConstraintForce=off  SenseConstraintForceX=off  SenseConstraintForceY=off  SenseConstraintForceZ=off  SenseConstraintTorque=off  SenseConstraintTorqueX=off  SenseConstraintTorqueY=off  SenseConstraintTorqueZ=off  SenseTotalForce=off  SenseTotalForceX=off  SenseTotalForceY=off  SenseTotalForceZ=off  SenseTotalTorque=off  SenseTotalTorqueX=off  SenseTotalTorqueY=off  SenseTotalTorqueZ=off  CompositeWrenchDir=FollowerOnBase  CompositeWrenchFrame=BaseFrame  RxEquilibriumPosition=0  RxEquilibriumPositionUnits=deg  RxSpringStiffness=0  RxSpringStiffnessUnits=N*m/deg  RxDampingCoefficient=0  RxDampingCoefficientUnits=N*m/(deg/s)  RxTorqueActuationMode=NoTorque  RxMotionActuationMode=ComputedMotion  RxSensePosition=on  RxSenseVelocity=on  RxSenseAcceleration=off  RxSenseTorqueForce=off  RxSenseLowerLimitTorqueForce=off  RxSenseUpperLimitTorqueForce=off  RxLowerLimitSpecify=off  RxLowerLimitBound=-90  RxLowerLimitBoundUnits=deg  RxLowerLimitStiffness=1e4  RxLowerLimitStiffnessUnits=N*m/deg  RxLowerLimitDamping=10  RxLowerLimitDampingUnits=N*m/(deg/s)  RxLowerLimitTransitionRegionWidth=0.1  RxLowerLimitTransitionRegionWidthUnits=deg  RxUpperLimitSpecify=off  RxUpperLimitBound=90  RxUpperLimitBoundUnits=deg  RxUpperLimitStiffness=1e4  RxUpperLimitStiffnessUnits=N*m/deg  RxUpperLimitDamping=10  RxUpperLimitDampingUnits=N*m/(deg/s)  RxUpperLimitTransitionRegionWidth=0.1  RxUpperLimitTransitionRegionWidthUnits=deg  RxPositionTargetSpecify=off  RxPositionTargetPriority=High  RxPositionTargetValue=0  RxPositionTargetValueUnits=deg  RxVelocityTargetSpecify=off  RxVelocityTargetPriority=High  RxVelocityTargetValue=0  RxVelocityTargetValueUnits=deg/s  RyEquilibriumPosition=0  RyEquilibriumPositionUnits=deg  RySpringStiffness=0  RySpringStiffnessUnits=N*m/deg  RyDampingCoefficient=0  RyDampingCoefficientUnits=N*m/(deg/s)  RyTorqueActuationMode=NoTorque  RyMotionActuationMode=ComputedMotion  RySensePosition=on  RySenseVelocity=on  RySenseAcceleration=off  RySenseTorqueForce=off  RySenseLowerLimitTorqueForce=off  RySenseUpperLimitTorqueForce=off  RyLowerLimitSpecify=off  RyLowerLimitBound=-90  RyLowerLimitBoundUnits=deg  RyLowerLimitStiffness=1e4  RyLowerLimitStiffnessUnits=N*m/deg  RyLowerLimitDamping=10  RyLowerLimitDampingUnits=N*m/(deg/s)  RyLowerLimitTransitionRegionWidth=0.1  RyLowerLimitTransitionRegionWidthUnits=deg  RyUpperLimitSpecify=off  RyUpperLimitBound=90  RyUpperLimitBoundUnits=deg  RyUpperLimitStiffness=1e4  RyUpperLimitStiffnessUnits=N*m/deg  RyUpperLimitDamping=10  RyUpperLimitDampingUnits=N*m/(deg/s)  RyUpperLimitTransitionRegionWidth=0.1  RyUpperLimitTransitionRegionWidthUnits=deg  RyPositionTargetSpecify=off  RyPositionTargetPriority=High  RyPositionTargetValue=0  RyPositionTargetValueUnits=deg  RyVelocityTargetSpecify=off  RyVelocityTargetPriority=High  RyVelocityTargetValue=0  RyVelocityTargetValueUnits=deg/s  RzEquilibriumPosition=0  RzEquilibriumPositionUnits=deg  RzSpringStiffness=0  RzSpringStiffnessUnits=N*m/deg  RzDampingCoefficient=0  RzDampingCoefficientUnits=N*m/(deg/s)  RzTorqueActuationMode=NoTorque  RzMotionActuationMode=ComputedMotion  RzSensePosition=on  RzSenseVelocity=on  RzSenseAcceleration=off  RzSenseTorqueForce=off  RzSenseLowerLimitTorqueForce=off  RzSenseUpperLimitTorqueForce=off  RzLowerLimitSpecify=off  RzLowerLimitBound=-90  RzLowerLimitBoundUnits=deg  RzLowerLimitStiffness=1e4  RzLowerLimitStiffnessUnits=N*m/deg  RzLowerLimitDamping=10  RzLowerLimitDampingUnits=N*m/(deg/s)  RzLowerLimitTransitionRegionWidth=0.1  RzLowerLimitTransitionRegionWidthUnits=deg  RzUpperLimitSpecify=off  RzUpperLimitBound=90  RzUpperLimitBoundUnits=deg  RzUpperLimitStiffness=1e4  RzUpperLimitStiffnessUnits=N*m/deg  RzUpperLimitDamping=10  RzUpperLimitDampingUnits=N*m/(deg/s)  RzUpperLimitTransitionRegionWidth=0.1  RzUpperLimitTransitionRegionWidthUnits=deg  RzPositionTargetSpecify=off  RzPositionTargetPriority=High  RzPositionTargetValue=0  RzPositionTargetValueUnits=deg  RzVelocityTargetSpecify=off  RzVelocityTargetPriority=High  RzVelocityTargetValue=0  RzVelocityTargetValueUnits=deg/s
  PS-S-{1,3,5..9} (7 alike) : nesl_utility/PS-Simulink Converter  PhysicalDomain=network_engine_domain  SubClassName=ps_output  LeftPortType=input  RightPortType=output  PseudoPeriodic=off  Frequencies=[]  Unit=1  AffineConversion=off
  PS-Simulink Converter1 : nesl_utility/PS-Simulink Converter  PhysicalDomain=network_engine_domain  SubClassName=ps_output  LeftPortType=input  RightPortType=output  PseudoPeriodic=off  Frequencies=[]  Unit=1  AffineConversion=off
  PS-Simulink Converter2 : nesl_utility/PS-Simulink Converter  PhysicalDomain=network_engine_domain  SubClassName=ps_output  LeftPortType=input  RightPortType=output  PseudoPeriodic=off  Frequencies=[]  Unit=1  AffineConversion=off
  Rigid Transform : sm_lib/Frames and Transforms/Rigid Transform  TranslationMethod=Cartesian  TranslationStandardOffset=0  TranslationLengthUnit=m  TranslationStandardAxis=+Z  TranslationCartesianOffset=[0 0 0.05]  TranslationROffset=0  TranslationROffsetUnits=m  TranslationZOffset=0  TranslationZOffsetUnits=m  TranslationThetaOffset=0  TranslationThetaOffsetUnits=deg  RotationMethod=StandardAxis  RotationAngleUnits=deg  RotationStandardAxis=+Z  RotationAngle=0.0  RotationArbitraryAxis=[0 0 1]  FollAlignAxisA=+X  BaseAlignAxisA=+Y  FollAlignAxisB=+Y  BaseAlignAxisB=+Z  RotationSequenceAxes=FollowerAxes  RotationSequence=XYX  RotationSequenceAngles=[0 0 0]  RotationSequenceAnglesUnits=deg  RotationMatrix=[1 0 0; 0 1 0; 0 0 1]
  Simulink-PS Converter1 : nesl_utility/Simulink-PS Converter  PhysicalDomain=network_engine_domain  SubClassName=ps_input  LeftPortType=input  RightPortType=output  PseudoPeriodic=off  Frequencies=[]  NoiseDistribution=none  NoiseParameters=[]  Unit=1  AffineConversion=off  FilteringAndDerivatives=zero  SimscapeFilterOrder=1  InputFilterTimeConstant=0.001  UdotUserProvided=1
  platform : PMIOPort  Side=Right
  ground : PMIOPort  Port=2  Side=Left
  Drone z-pos : Outport  VectorParamsAs1DForOutWhenUnconnected=off
  z-vel : Outport  Port=2  VectorParamsAs1DForOutWhenUnconnected=off
  x-pos : Outport  Port=3  VectorParamsAs1DForOutWhenUnconnected=off
  x-vel : Outport  Port=4  VectorParamsAs1DForOutWhenUnconnected=off
  y-pos : Outport  Port=5  VectorParamsAs1DForOutWhenUnconnected=off
  y-vel : Outport  Port=6  VectorParamsAs1DForOutWhenUnconnected=off
  x-roll : Outport  Port=7  VectorParamsAs1DForOutWhenUnconnected=off
  y-pitch : Outport  Port=8  VectorParamsAs1DForOutWhenUnconnected=off
  z-yaw : Outport  Port=9  VectorParamsAs1DForOutWhenUnconnected=off
  wires:
  Dæmpet understel/1(Ground_N) -> Simulink-PS Converter1/1
  PS-Simulink Converter1/1 -> Drone z-pos/1, Dæmpet understel/2(Height)
  PS-Simulink Converter2/1 -> Dæmpet understel/1(Heingt_rate), z-vel/1
  PS-S-6/1 -> x-pos/1
  PS-S-7/1 -> x-vel/1
  PS-S-8/1 -> y-pos/1
  PS-S-9/1 -> y-vel/1
  PS-S-1/1 -> x-roll/1
  PS-S-3/1 -> y-pitch/1
  PS-S-5/1 -> z-yaw/1
  connections:
  Rigid Transform/LConn1 -- ground/RConn1
  Simulink-PS Converter1/RConn1 -- Cartesian Joint/LConn2
  PS-Simulink Converter1/LConn1 -- Cartesian Joint/RConn6
  PS-Simulink Converter2/LConn1 -- Cartesian Joint/RConn7
  platform/RConn1 -- Gimbal Joint/RConn1
  PS-S-6/LConn1 -- Cartesian Joint/RConn2
  PS-S-7/LConn1 -- Cartesian Joint/RConn3
  PS-S-8/LConn1 -- Cartesian Joint/RConn4
  PS-S-9/LConn1 -- Cartesian Joint/RConn5
  Cartesian Joint/LConn1 -- Rigid Transform/RConn1
  Gimbal Joint/LConn1 -- Cartesian Joint/RConn1
  PS-S-1/LConn1 -- Gimbal Joint/RConn2
  PS-S-3/LConn1 -- Gimbal Joint/RConn4
  PS-S-5/LConn1 -- Gimbal Joint/RConn6

== system simulink_tri_motor_drone/Height reg/Coarse controller (>5m error) ==
  fejl : Inport
  Action Port : ActionPort  ActionPortLabel=if(u1 > 5)
  KD1 : Constant  Value=KDheightcoarse
  KI1 : Constant  Value=KIheightcoarse
  KP1 : Constant  Value=KPheightcoarse
  height-controller-coarse : Subsystem
  u-trust1 : Outport  VectorParamsAs1DForOutWhenUnconnected=off
  wires:
  KI1/1 -> height-controller-coarse/1(KI)
  KP1/1 -> height-controller-coarse/3(KP)
  KD1/1 -> height-controller-coarse/2(KD)
  height-controller-coarse/1(Out1) -> u-trust1/1
  fejl/1 -> height-controller-coarse/4(fejl)

== system simulink_tri_motor_drone/Height reg/Fine controller (<5m error) ==
  fejl : Inport
  Action Port : ActionPort  ActionPortLabel=else
  Constant : Constant  Value=hoverVoltagefine
  KD : Constant  Value=KDheightfine
  KI : Constant  Value=KIheightfine
  KP : Constant  Value=KPheightfine
  Sum : Sum  Inputs=|++
  height-controller-fine : Subsystem
  u-trust : Outport  VectorParamsAs1DForOutWhenUnconnected=off
  wires:
  fejl/1 -> height-controller-fine/4(fejl)
  KI/1 -> height-controller-fine/1(KI)
  KP/1 -> height-controller-fine/3(KP)
  KD/1 -> height-controller-fine/2(KD)
  Sum/1 -> u-trust/1
  Constant/1 -> Sum/2
  height-controller-fine/1(Out1) -> Sum/1

== system simulink_tri_motor_drone/Height reg/height-controller-fine ==
  KI : Inport
  KD : Inport  Port=2
  KP : Inport  Port=3
  fejl : Inport  Port=4
  Delay : Delay  DelayLength=1  InitialCondition=0  SampleTime=Ts
  Delay1 : Delay  DelayLength=1  InitialCondition=0  SampleTime=Ts
  Divide : Product  Inputs=*/
  Product{,1..3} (4 alike) : Product
  Saturation : Saturate  UpperLimit=0.3  LowerLimit=-0.3
  Sum2 : Sum  Inputs=|-+
  Sum3 : Sum  Inputs=|++
  Sum4 : Sum  Inputs=+|++
  Zero-Order Hold : ZeroOrderHold  SampleTime=Ts
  height-D-term : Scope
  height-integrator : Scope
  sample-frq : Constant  Value=1/Ts
  Out1 : Outport  VectorParamsAs1DForOutWhenUnconnected=off
  wires:
  fejl/1 -> Zero-Order Hold/1
  sample-frq/1 -> Divide/2, Product/2
  Product3/1 -> Product1/2, Product2/1, Sum4/1
  Zero-Order Hold/1 -> Product3/2
  Divide/1 -> Sum3/1
  Sum2/1 -> Product/1
  KD/1 -> Product1/1
  KP/1 -> Product3/1
  Sum3/1 -> Saturation/1
  Delay/1 -> Sum2/1
  Delay1/1 -> Sum3/2
  Sum4/1 -> Out1/1
  Saturation/1 -> Sum4/2, Delay1/1, height-integrator/1
  Product/1 -> height-D-term/1, Sum4/3
  Product2/1 -> Divide/1
  KI/1 -> Product2/2
  Product1/1 -> Sum2/2, Delay/1

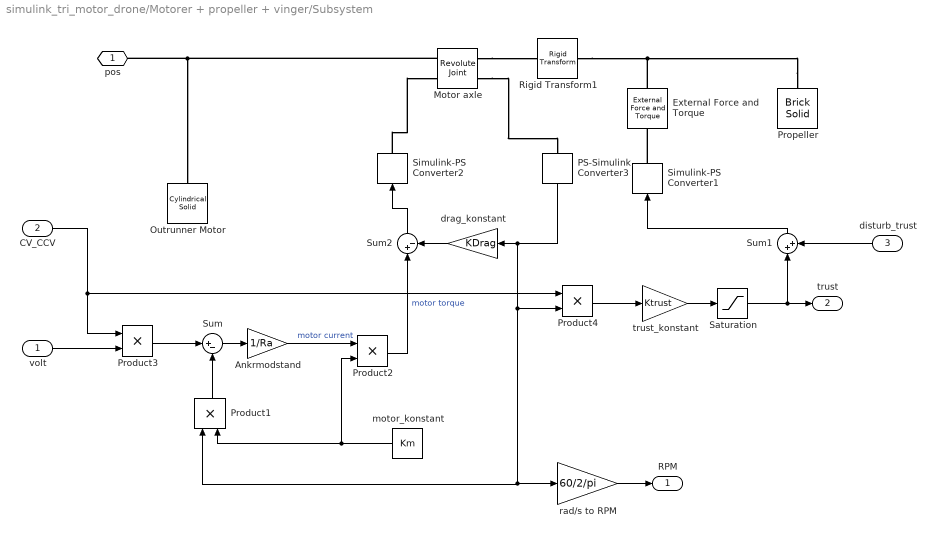
== system simulink_tri_motor_drone/Motorer + propeller + vinger/Subsystem ==
  volt : Inport
  CV_CCV : Inport  Port=2
  disturb_trust : Inport  Port=3
  Ankrmodstand : Gain  Gain=1/Ra
  External Force and Torque : sm_lib/Forces and Torques/External Force and Torque  ForceResolutionFrame=AttachedFrame  EnableForceX=off  EnableForceY=off  EnableForceZ=on  EnableForce=off  TorqueResolutionFrame=AttachedFrame  EnableTorqueX=off  EnableTorqueY=off  EnableTorqueZ=off  EnableTorque=off
  Motor axle : sm_lib/Joints/Revolute Joint  JointMode=Normal  SenseConstraintForce=off  SenseConstraintForceX=off  SenseConstraintForceY=off  SenseConstraintForceZ=off  SenseConstraintTorque=off  SenseConstraintTorqueX=off  SenseConstraintTorqueY=off  SenseConstraintTorqueZ=off  SenseTotalForce=off  SenseTotalForceX=off  SenseTotalForceY=off  SenseTotalForceZ=off  SenseTotalTorque=off  SenseTotalTorqueX=off  SenseTotalTorqueY=off  SenseTotalTorqueZ=off  CompositeWrenchDir=FollowerOnBase  CompositeWrenchFrame=BaseFrame  EquilibriumPosition=0  EquilibriumPositionUnits=deg  SpringStiffness=0  SpringStiffnessUnits=N*m/deg  DampingCoefficient=0  DampingCoefficientUnits=N*m/(deg/s)  TorqueActuationMode=InputTorque  MotionActuationMode=ComputedMotion  SensePosition=off  SenseVelocity=on  SenseAcceleration=off  SenseTorqueForce=off  SenseLowerLimitTorqueForce=off  SenseUpperLimitTorqueForce=off  LowerLimitSpecify=off  LowerLimitBound=-90  LowerLimitBoundUnits=deg  LowerLimitStiffness=1e4  LowerLimitStiffnessUnits=N*m/deg  LowerLimitDamping=10  LowerLimitDampingUnits=N*m/(deg/s)  LowerLimitTransitionRegionWidth=0.1  LowerLimitTransitionRegionWidthUnits=deg  UpperLimitSpecify=off  UpperLimitBound=90  UpperLimitBoundUnits=deg  UpperLimitStiffness=1e4  UpperLimitStiffnessUnits=N*m/deg  UpperLimitDamping=10  UpperLimitDampingUnits=N*m/(deg/s)  UpperLimitTransitionRegionWidth=0.1  UpperLimitTransitionRegionWidthUnits=deg  PositionTargetSpecify=off  PositionTargetPriority=High  PositionTargetValue=0  PositionTargetValueUnits=deg  VelocityTargetSpecify=on  VelocityTargetPriority=High  VelocityTargetValue=-hoverVel  VelocityTargetValueUnits=rad/s
  Outrunner Motor : sm_lib/Body Elements/Cylindrical Solid  GraphicAmbientColor=[0.15 0.15 0.15 1.0]  BasedOnType=Mass  CenterOfMass=[0 0 0]  CenterOfMassUnits=m  GraphicDiffuseColor=[1.0 0.8 0.0]  CylinderLength=0.05  CylinderLengthUnits=m  CylinderRadius=0.01  CylinderRadiusUnits=m  Density=1000  DensityUnits=kg/(m^3)  DoExposeReferenceFrame=on  GraphicEmissiveColor=[0.0 0.0 0.0 1.0]  ExportEntireGeometry=off  SerializedFrames=<Frames/>  MarkerShape=Sphere  MarkerSize=10  GraphicType=FromGeometry  InertiaType=CalculateFromGeometry  Mass=motorMass  MassUnits=kg  MomentsOfInertia=[1 1 1]  MomentsOfInertiaUnits=kg*m^2  GraphicOpacity=1.0  ProductsOfInertia=[0 0 0]  ProductsOfInertiaUnits=kg*m^2  GraphicShininess=75  GraphicSpecularColor=[0.5 0.5 0.5 1.0]  GraphicVisPropType=SimpleVisualProperties
  PS-Simulink Converter3 : nesl_utility/PS-Simulink Converter  PhysicalDomain=network_engine_domain  SubClassName=ps_output  LeftPortType=input  RightPortType=output  PseudoPeriodic=off  Frequencies=[]  Unit=1  AffineConversion=off
  Product{1..4} (4 alike) : Product
  Propeller : sm_lib/Body Elements/Brick Solid  GraphicAmbientColor=[0.15 0.15 0.15 1.0]  BasedOnType=Mass  BrickDimensions=[0.2 0.03 0.01]  BrickDimensionUnits=m  CenterOfMass=[0 0 0]  CenterOfMassUnits=m  GraphicDiffuseColor=[1.0 0.8 0.0]  Density=1000  DensityUnits=kg/(m^3)  DoExposeReferenceFrame=on  GraphicEmissiveColor=[0.0 0.0 0.0 1.0]  ExportEntireGeometry=off  SerializedFrames=<Frames/>  MarkerShape=Sphere  MarkerSize=10  GraphicType=FromGeometry  InertiaType=CalculateFromGeometry  Mass=propellerMass  MassUnits=kg  MomentsOfInertia=[1 1 1]  MomentsOfInertiaUnits=kg*m^2  GraphicOpacity=1.0  ProductsOfInertia=[0 0 0]  ProductsOfInertiaUnits=kg*m^2  GraphicShininess=75  GraphicSpecularColor=[0.5 0.5 0.5 1.0]  GraphicVisPropType=SimpleVisualProperties
  Rigid Transform1 : sm_lib/Frames and Transforms/Rigid Transform  TranslationMethod=Cartesian  TranslationStandardOffset=0  TranslationLengthUnit=m  TranslationStandardAxis=+Z  TranslationCartesianOffset=[0 0 0.03]  TranslationROffset=0  TranslationROffsetUnits=m  TranslationZOffset=0  TranslationZOffsetUnits=m  TranslationThetaOffset=0  TranslationThetaOffsetUnits=deg  RotationMethod=StandardAxis  RotationAngleUnits=deg  RotationStandardAxis=+Z  RotationAngle=0.0  RotationArbitraryAxis=[0 0 1]  FollAlignAxisA=+X  BaseAlignAxisA=+Y  FollAlignAxisB=+Y  BaseAlignAxisB=+Z  RotationSequenceAxes=FollowerAxes  RotationSequence=XYX  RotationSequenceAngles=[0 0 0]  RotationSequenceAnglesUnits=deg  RotationMatrix=[1 0 0; 0 1 0; 0 0 1]
  Saturation : Saturate  UpperLimit=inf  LowerLimit=0
  Simulink-PS Converter1 : nesl_utility/Simulink-PS Converter  PhysicalDomain=network_engine_domain  SubClassName=ps_input  LeftPortType=input  RightPortType=output  PseudoPeriodic=off  Frequencies=[]  NoiseDistribution=none  NoiseParameters=[]  Unit=1  AffineConversion=off  FilteringAndDerivatives=zero  SimscapeFilterOrder=1  InputFilterTimeConstant=0.001  UdotUserProvided=1
  Simulink-PS Converter2 : nesl_utility/Simulink-PS Converter  PhysicalDomain=network_engine_domain  SubClassName=ps_input  LeftPortType=input  RightPortType=output  PseudoPeriodic=off  Frequencies=[]  NoiseDistribution=none  NoiseParameters=[]  Unit=1  AffineConversion=off  FilteringAndDerivatives=zero  SimscapeFilterOrder=1  InputFilterTimeConstant=0.001  UdotUserProvided=1
  Sum : Sum  Inputs=|+-
  Sum1 : Sum  Inputs=|++
  Sum2 : Sum  Inputs=|+-
  drag_konstant : Gain  Gain=KDrag
  motor_konstant : Constant  Value=Km
  rad/s to RPM : Gain  Gain=60/2/pi
  trust_konstant : Gain  Gain=Ktrust
  pos : PMIOPort  Side=Left
  RPM : Outport  VectorParamsAs1DForOutWhenUnconnected=off
  trust : Outport  Port=2  VectorParamsAs1DForOutWhenUnconnected=off
  wires:
  PS-Simulink Converter3/1 -> Product4/2, Product1/1, rad/s to RPM/1, drag_konstant/1
  drag_konstant/1 -> Sum2/2
  Product1/1 -> Sum/2
  trust_konstant/1 -> Saturation/1
  Product2/1 -> Sum2/1  "motor torque"
  disturb_trust/1 -> Sum1/2
  Sum/1 -> Ankrmodstand/1
  Sum2/1 -> Simulink-PS Converter2/1
  Ankrmodstand/1 -> Product2/1  "motor current"
  motor_konstant/1 -> Product1/2, Product2/2
  rad/s to RPM/1 -> RPM/1
  volt/1 -> Product3/2
  Product3/1 -> Sum/1
  Sum1/1 -> Simulink-PS Converter1/1
  CV_CCV/1 -> Product4/1, Product3/1
  Product4/1 -> trust_konstant/1
  Saturation/1 -> trust/1, Sum1/1
  connections:
  pos/RConn1 -- Motor axle/LConn1 -- Outrunner Motor/RConn1
  Propeller/RConn1 -- Rigid Transform1/RConn1 -- External Force and Torque/RConn1
  Simulink-PS Converter2/RConn1 -- Motor axle/LConn2
  Motor axle/RConn1 -- Rigid Transform1/LConn1
  Motor axle/RConn2 -- PS-Simulink Converter3/LConn1
  Simulink-PS Converter1/RConn1 -- External Force and Torque/LConn1
